simulink model "MyUserDriver_RTW"  (Simulink 10.3)
settings: Solver=ode1  StartTime=0.0  StopTime=inf  FixedStep=0.001  RelTol=1e-3
PreLoadFcn:
  | vehicle = 'Car'; if ~length(which('cmself')), cmenv; end
  | MyUserDriver_RTW_bus;
  | MyUserDriver_RTW_params;
InitFcn:
  | vehicle = 'Car'; if ~length(which('cmself')), cmenv; end
  | MyUserDriver_RTW_bus
undefined symbols (not defined in the file): kd, ki, kp, TLPF, tPrev, vTrgt
libraries: CarMaker4SL x2, simulink x1
Description:
  | CarMaker Plug-in Model Target
settings Model: Creator=IPG  LastModifiedBy=IPG  MultithreadedSim=on
settings DataIOCC: SaveFormat=Dataset  SignalLoggingSaveFormat=Dataset
settings OptimizationCC: ExpressionDepthLimit=128  LifeSpan=auto
settings DebuggingCC: UnderspecifiedInitializationDetection=Simplified  MergeDetectMultiDrivingBlocksExec=error  FcnCallInpInsideContextMsg=error  StateNameClashWarn=none  PregeneratedLibrarySubsystemCodeDiagnostic=none  SFUnexpectedBacktrackingDiag=error  SFNoUnconditionalDefaultTransitionDiag=error  SFExecutionAtInitializationDiag=warning
settings HardwareCC: ProdBitPerPointer=64  ProdBitPerSizeT=64  ProdBitPerPtrDiffT=64  ProdLargestAtomicFloat=Float  ProdIntDivRoundTo=Zero  ProdEndianess=LittleEndian  ProdWordSize=64  ProdHWDeviceType=Intel->x86-64 (Windows64)
settings ModelReferenceCC: PropagateSignalLabelsOutOfModel=on
settings RTWCC: Description=CarMaker Plug-in Model Target  SystemTargetFile=CarMaker.tlc  TemplateMakefile=CarMaker_unix-linux64.tmf
settings CodeAppCC: MaxIdLength=127  StateflowObjectComments=off
settings STFCustomTargetCC: TargetLangStandard=C99 (ISO)  CombineOutputUpdateFcns=on  CodeInterfacePackaging=Reusable function  GRTInterface=off  GenerateAllocFcn=on  SystemTargetFile=CarMaker.tlc
settings GRTTargetCC: TargetLangStandard=C99 (ISO)  ParMdlRefBuildCompliant=off  CompOptLevelCompliant=off  ConcurrentExecutionCompliant=off  CombineOutputUpdateFcns=on  MatFileLogging=off  CodeInterfacePackaging=Reusable function  CPPClassGenCompliant=off  GRTInterface=off  GenerateAllocFcn=on  UseToolchainInfoCompliant=off
settings CustomProperty: DataType=string
settings EnumStrPairs: String=Car
settings ConfigComp: CovMetricSettings=dwe  CovSaveCumulativeToWorkspaceVar=off  CovSaveSingleToWorkspaceVar=off  CovExternalEMLEnable=on

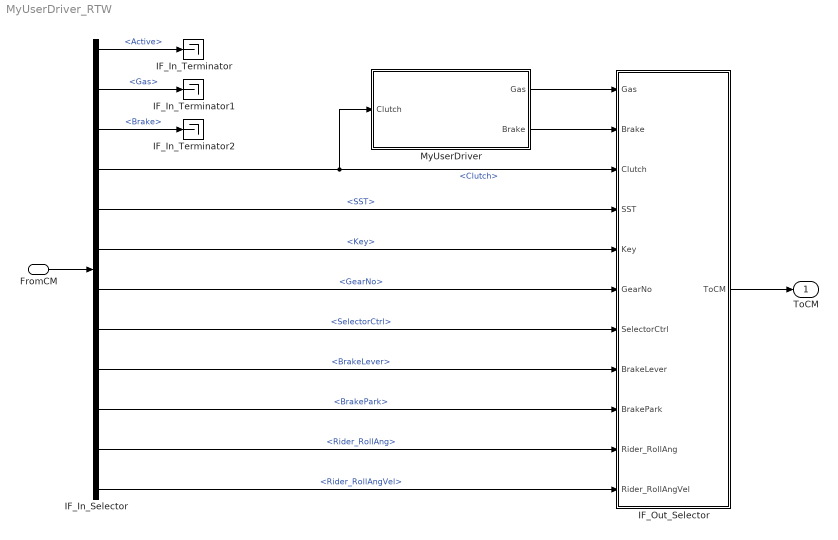
== system MyUserDriver_RTW ==
  FromCM : Inport  OutDataTypeStr=Bus: cmUserDriverIn
  IF_In_Selector : BusSelector  OutputSignals=Active,Gas,Brake,Clutch,SST,Key,GearNo,SelectorCtrl,BrakeLever,BrakePark,Rider_RollAng,Rider_RollAngVel
  IF_In_Terminator : Terminator
  IF_In_Terminator1 : Terminator
  IF_In_Terminator2 : Terminator
  IF_Out_Selector : Subsystem  mask(Signal Selection){}
      mask help: Signal Selection Block
      settings: OpenFcn=cmSignalSelect('SignalSelection_CB',gcb)
  MyUserDriver : Subsystem
  ToCM : Outport  OutDataTypeStr=Bus: cmUserDriverOut  VectorParamsAs1DForOutWhenUnconnected=off
  wires:
  FromCM/1 -> IF_In_Selector/1
  IF_Out_Selector/1(ToCM) -> ToCM/1
  MyUserDriver/2(Brake) -> IF_Out_Selector/2(Brake)
  MyUserDriver/1(Gas) -> IF_Out_Selector/1(Gas)
  IF_In_Selector/5 -> IF_Out_Selector/4(SST)  "<SST>"
  IF_In_Selector/6 -> IF_Out_Selector/5(Key)  "<Key>"
  IF_In_Selector/7 -> IF_Out_Selector/6(GearNo)  "<GearNo>"
  IF_In_Selector/8 -> IF_Out_Selector/7(SelectorCtrl)  "<SelectorCtrl>"
  IF_In_Selector/9 -> IF_Out_Selector/8(BrakeLever)  "<BrakeLever>"
  IF_In_Selector/10 -> IF_Out_Selector/9(BrakePark)  "<BrakePark>"
  IF_In_Selector/4 -> MyUserDriver/1(Clutch), IF_Out_Selector/3(Clutch)  "<Clutch>"
  IF_In_Selector/11 -> IF_Out_Selector/10(Rider_RollAng)  "<Rider_RollAng>"
  IF_In_Selector/12 -> IF_Out_Selector/11(Rider_RollAngVel)  "<Rider_RollAngVel>"
  IF_In_Selector/3 -> IF_In_Terminator2/1  "<Brake>"
  IF_In_Selector/2 -> IF_In_Terminator1/1  "<Gas>"
  IF_In_Selector/1 -> IF_In_Terminator/1  "<Active>"

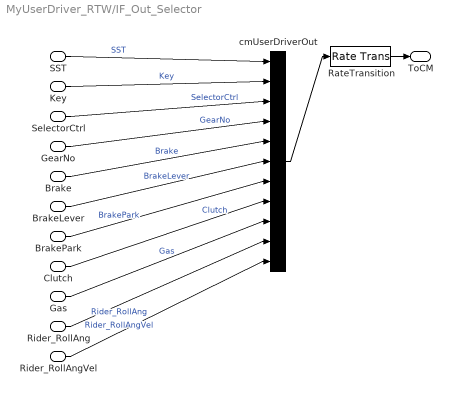
== system MyUserDriver_RTW/IF_Out_Selector ==
  Gas : Inport
  Brake : Inport  Port=2
  Clutch : Inport  Port=3
  SST : Inport  Port=4
  Key : Inport  Port=5
  GearNo : Inport  Port=6
  SelectorCtrl : Inport  Port=7
  BrakeLever : Inport  Port=8
  BrakePark : Inport  Port=9
  Rider_RollAng : Inport  Port=10
  Rider_RollAngVel : Inport  Port=11
  RateTransition : RateTransition  OutPortSampleTime=str2num(get_param(bdroot,'FixedStep'))
  cmUserDriverOut : BusCreator  Inputs=11
  ToCM : Outport  VectorParamsAs1DForOutWhenUnconnected=off
  wires:
  RateTransition/1 -> ToCM/1
  cmUserDriverOut/1 -> RateTransition/1
  Gas/1 -> cmUserDriverOut/9  "Gas"
  Brake/1 -> cmUserDriverOut/5  "Brake"
  SST/1 -> cmUserDriverOut/1  "SST"
  Key/1 -> cmUserDriverOut/2  "Key"
  SelectorCtrl/1 -> cmUserDriverOut/3  "SelectorCtrl"
  GearNo/1 -> cmUserDriverOut/4  "GearNo"
  BrakeLever/1 -> cmUserDriverOut/6  "BrakeLever"
  BrakePark/1 -> cmUserDriverOut/7  "BrakePark"
  Clutch/1 -> cmUserDriverOut/8  "Clutch"
  Rider_RollAng/1 -> cmUserDriverOut/10  "Rider_RollAng"
  Rider_RollAngVel/1 -> cmUserDriverOut/11  "Rider_RollAngVel"

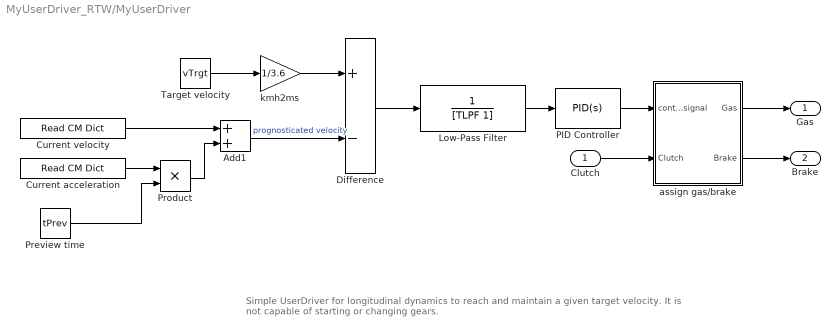
== system MyUserDriver_RTW/MyUserDriver ==
  note: Simple UserDriver for longitudinal dynamics to reach and maintain a given
      | target velocity. It is not capable of starting or changing gears.
  Clutch : Inport
  Add1 : Sum
  Current acceleration : CarMaker4SL/Read CM Dict  xname=Vhcl.PoI.ax_1  xsync=off  xstime=Continuous
  Current velocity : CarMaker4SL/Read CM Dict  xname=Vhcl.PoI.vx_1  xsync=off  xstime=Continuous
  Difference : Sum  Inputs=+-
  Low-Pass Filter : TransferFcn  Denominator=[TLPF 1]
  PID Controller : simulink/Continuous/PID Controller  Controller=PID  Form=Parallel  TimeDomain=Continuous-time  SampleTime=-1  IntegratorMethod=Forward Euler  FilterMethod=Forward Euler  ControllerParametersSource=internal  P=kp  I=ki  D=kd  UseFilter=on  N=100  TunerSelectOption=Transfer Function Based (PID Tuner App)  InitialConditionSource=internal  InitialConditionForIntegrator=0  InitialConditionForFilter=0  DifferentiatorICPrevScaledInput=0  ExternalReset=none  TrackingMode=off  Kt=1  LimitOutput=on  UpperSaturationLimit=1  LowerSaturationLimit=-1  LinearizeAsGain=on  AntiWindupMode=clamping  Kb=1  POutMin=[]  POutMax=[]  IOutMin=[]  IOutMax=[]  DOutMin=[]  DOutMax=[]  NOutMin=[]  NOutMax=[]  SumOutMin=[]  SumOutMax=[]  SaturationOutMin=[]  SaturationOutMax=[]  PParamMin=[]  PParamMax=[]  IParamMin=[]  IParamMax=[]  DParamMin=[]  DParamMax=[]  NParamMin=[]  NParamMax=[]  KbParamMin=[]  KbParamMax=[]  KtParamMin=[]  KtParamMax=[]  KbOutMin=[]  KbOutMax=[]  KtOutMin=[]  KtOutMax=[]  IntegratorOutMin=[]  IntegratorOutMax=[]  FilterOutMin=[]  FilterOutMax=[]  SumI1OutMin=[]  SumI1OutMax=[]  SumI2OutMin=[]  SumI2OutMax=[]  SumI3OutMin=[]  SumI3OutMax=[]  SumDOutMin=[]  SumDOutMax=[]  DifferentiatorOutMin=[]  DifferentiatorOutMax=[]  FilterDiffOutCoefMin=[]  FilterDiffOutCoefMax=[]  ReciprocalOutMin=[]  ReciprocalOutMax=[]  SumDenOutMin=[]  SumDenOutMax=[]  SumNumOutMin=[]  SumNumOutMax=[]  DivideOutMin=[]  DivideOutMax=[]  IntegratorContinuousStateAttributes=''  IntegratorStateMustResolveToSignalObject=off  IntegratorRTWStateStorageClass=Auto  FilterContinuousStateAttributes=''  FilterStateMustResolveToSignalObject=off  FilterRTWStateStorageClass=Auto
  Preview time : Constant  Value=tPrev
  Product : Product
  Target velocity : Constant  Value=vTrgt
  assign gas/brake : Subsystem
  kmh2ms : Gain  Gain=1/3.6
  Gas : Outport  VectorParamsAs1DForOutWhenUnconnected=off
  Brake : Outport  Port=2  VectorParamsAs1DForOutWhenUnconnected=off
  wires:
  Current velocity/1 -> Add1/1
  Target velocity/1 -> kmh2ms/1
  PID Controller/1 -> assign gas/brake/1(control signal)
  assign gas/brake/1(Gas) -> Gas/1
  assign gas/brake/2(Brake) -> Brake/1
  Current acceleration/1 -> Product/1
  Product/1 -> Add1/2
  Preview time/1 -> Product/2
  Add1/1 -> Difference/2  "prognosticated velocity"
  Low-Pass Filter/1 -> PID Controller/1
  Clutch/1 -> assign gas/brake/2(Clutch)
  Difference/1 -> Low-Pass Filter/1
  kmh2ms/1 -> Difference/1

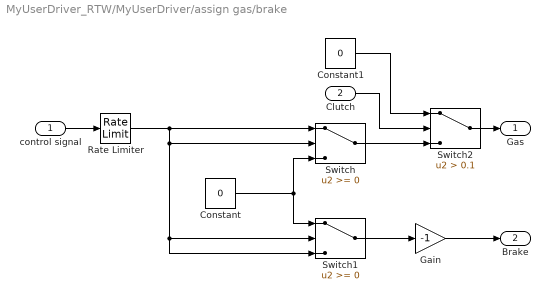
== system MyUserDriver_RTW/MyUserDriver/assign gas/brake ==
  control signal : Inport
  Clutch : Inport  Port=2
  Constant : Constant  Value=0
  Constant1 : Constant  Value=0
  Gain : Gain  Gain=-1
  Rate Limiter : RateLimiter  SampleTimeMode=inherited
  Switch : Switch
  Switch1 : Switch
  Switch2 : Switch  Criteria=u2 > Threshold  Threshold=0.1
  Gas : Outport  VectorParamsAs1DForOutWhenUnconnected=off
  Brake : Outport  Port=2  VectorParamsAs1DForOutWhenUnconnected=off
  wires:
  Switch1/1 -> Gain/1
  Rate Limiter/1 -> Switch1/2, Switch1/3, Switch/2, Switch/1
  Constant/1 -> Switch1/1, Switch/3
  Switch/1 -> Switch2/3
  Gain/1 -> Brake/1
  control signal/1 -> Rate Limiter/1
  Clutch/1 -> Switch2/2
  Constant1/1 -> Switch2/1
  Switch2/1 -> Gas/1
